simulink model "psbturbine"  (Simulink 6.0)
settings: Solver=ode23tb  SolverMode=SingleTasking  StartTime=0.0  StopTime=2  RelTol=1e-3
undefined symbols (not defined in the file or in its folder): D1, Delta
libraries: powerlib2 x15
settings Model: Creator=patrice  LastModifiedBy=batserve  ExtModeTrigMode=oneshot  ExtModeArmWhenConnect=off  ExtModeAutoUpdateStatusClock=off
settings DataIOCC: LimitDataPoints=off  SignalLoggingName=sigsOut
settings OptimizationCC: BlockReduction=off  BooleanDataType=off
settings DebuggingCC: CheckExecutionContextPreStartOutputMsg=on  CheckExecutionContextRuntimeOutputMsg=on  SolverPrmCheckMsg=none
settings HardwareCC: TargetUnknown=on
settings RTWCC: TemplateMakefile=grt_unix.tmf

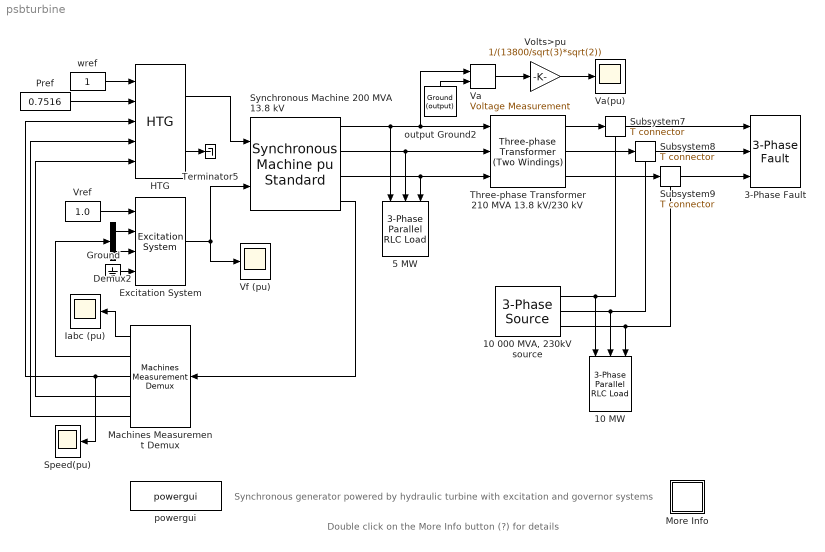
== system psbturbine ==
  note: Double click on the More Info button (?) for details
  note: Synchronous generator powered by hydraulic turbine
      |  with excitation and governor systems
  " Iabc (pu)" : Scope
      settings: TickLabels=on  TimeRange=0.2  YMax=6  DataFormat=Array
  " Speed(pu)" : Scope
      settings: TickLabels=on  TimeRange=2  YMin=0.98  YMax=1.02  SaveName=Pm  DataFormat=Array
  "10 000 MVA, 230kV source" : powerlib2/Electrical Sources/3-Phase Source  Tag=PoWeRsYsTeMbLoCk  V=230e3  Phi=0  F=60  InternalConnection=Yg  RLoff=on  R=0.529  L=0.0140  Psc=10000e6  Vbase=230e3  XRratio=10  PSBOutputType=111
  10 MW : powerlib2/Elements/3-Phase Parallel RLC Load  Orientation=down  Vpp=230e3  fn=60  P3=10e6  QL3=0  QC3=0
  3-Phase Fault : powerlib2/Elements/3-Phase Fault  sa=on  sb=on  sc=on  Rdef=1e-3  st=on  Rt=1e-3  comext=off  sw_status=[1 0]  sw_times=[ 0.1 0.2]  Ts=0  init_statext=[1 1 0]  Rp=inf  Cp=inf  mesure=None
  5 MW : powerlib2/Elements/3-Phase Parallel RLC Load  Orientation=down  Vpp=13.8e3  fn=60  P3=5e6  QL3=0  QC3=0
  Demux2 : Demux  Outputs=2
  Excitation System : powerlib2/Machines/Excitation System  tr=20e-3  reg=[ 300, 0.001 ]  exc=[ 1, 0 ]  tgr=[ 0, 0 ]  damp=[ 0.001, 0.1 ]  sat=[ 0, 0 ]  lim=[ -11.5, 11.5, 0 ]  v0=[1,1.0]
  Ground : Ground
  HTG : powerlib2/Machines/HTG  sm="[ 10/3  0.07 ]"  gate="[  0.01  0.97518  -0.1  0.1 ]"  reg="[  0.05  1.163  0.105  0  0.01  ]"  hyd="[  0  2.67  ]"  dref=0  po=1
  Machines Measurement Demux : powerlib2/Machines/Machines Measurement Demux  Orientation=left  machType=Synchronous  ssm1=on  ssm2=on  ssm3=on  ssm4=on  ssm5=on  ssm6=on  sm1=on  sm2=off  sm3=off  sm4=off  sm5=off  sm6=on  sm7=off  sm8=on  sm9=off  sm10=on  sm11=off  sm115=off  sm12=off  sm13=on  sm14=off  asm1=on  asm2=on  asm3=on  asm4=on  asm5=on  asm6=on  asm7=on  asm8=on  asm9=on  asm10=on  asm11=on  pmsm1=on  pmsm2=on  pmsm3=on  pmsm4=on  pmsm5=on  pmsm6=on  lastType=2
  More Info : Subsystem
      mask Display: disp('?')
  Pref : Constant  Value=0.7516
  Subsystem7 : powerlib2/Connectors/T connector  Tag=PoWeRsYsTeMbLoCk  PSBOutputType=1
  Subsystem8 : powerlib2/Connectors/T connector  Tag=PoWeRsYsTeMbLoCk  PSBOutputType=1
  Subsystem9 : powerlib2/Connectors/T connector  Tag=PoWeRsYsTeMbLoCk  PSBOutputType=1
  Synchronous Machine 200 MVA 13.8 kV : powerlib2/Machines/Synchronous Machine pu Standard  Tag=PoWeRsYsTeMbLoCk  rotorType=Salient-pole  x1="[ 200E6  13800   60 ]"  x2b=[ 31 32 33 34 35 36 37 ]  x2=[ 1.305, 0.296, 0.252, 0.474, 0.243, 0.18 ]  dAxisT=Short-circuit  qAxisT=Open-circuit  x3a=[]  x3b=[]  x3c=[]  x3d=[]  x3=[ 1.01, 0.053, 0.1 ]  x3e=[]  x3f=[]  x3g=[]  x4=2.8544e-3  x5="[ 3.2 0  32]"  x6=[0 0 0 0 0 0 0 0 1]  x7=off  x8=[0.6404,0.7127,0.8441,0.9214,0.9956,1.082,1.19,1.316,1.457;0.7,0.7698,0.8872,0.9466,0.9969,1.046,1.1,1.151,1.201]  PSBOutputType=1110  iounits=0.5  LoadFlowParameters=[1 150000000 0 0]
  Terminator5 : Terminator
  Three-phase Transformer 210 MVA 13.8 kV/230 kV : powerlib2/Elements/Three-phase Transformer (Two Windings)  Tag=PoWeRsYsTeMbLoCk  nominal=[ 210e6 60 ]  type1=Delta (D1)  params1="[ 13.8e3 0.0027  0.08]"  type2=Yg  params2=[ 230e3 0.0027 0.08]  ynsat=off  rmag=500  lm=500  sat="[ 0,0  ;  0.005,1.2  ;  1.0,1.4 ]"  hyst=off  matfile='hysteresis'  sif=off  phi0=[ 0.8 , -0.8 , 0.7 ]  initialslopes=[+1 +1 +1]  mesure=None  PSBOutputType=1111
  Va : powerlib2/Measurements/Voltage Measurement  Tag=PoWeRsYsTeMmEaSuReMeNt  PhasorSimulation=off  OutputType=Magnitude  PSBOutputType=0  PSBequivalent=0
  Va(pu) : Scope
      settings: TickLabels=on  TimeRange=0.2  YMin=-1.25  YMax=1.25  SaveName=vf  DataFormat=Array
  Vf (pu) : Scope
      settings: TickLabels=on  TimeRange=2  YMin=-10  YMax=15  SaveName=vf  DataFormat=Array
  Volts>pu : Gain  Gain=1/(13800/sqrt(3)*sqrt(2))  SaturateOnIntegerOverflow=on
  Vref : Constant  Value=1.0
  output Ground2 : powerlib2/Connectors/Ground (output)  Tag=PoWeRsYsTeMbLoCk  Orientation=up  PSBOutputType=1
  powergui : powerlib2/powergui  Frange=logspace(0,3,50)  Ylog=off  Xlog=off  save=off  variable=ZData  ZoomFFT=on  StartTime=0.0  cycles=2  DisplayStyle=off  fundamental=60  FreqAxis=off  MaxFrequency=1000  frequencyindice=1  frequencyindicesteady=1  RmsSteady=1  display=off  Ts=0  methode=off  frequency=60  echomessages=off
  wref : Constant
  wires:
  Ground/1 -> Excitation System/4
  HTG/2 -> Terminator5/1
  Excitation System/1 -> Vf (pu)/1, Synchronous Machine 200 MVA 13.8 kV/2
  Vref/1 -> Excitation System/1
  HTG/1 -> Synchronous Machine 200 MVA 13.8 kV/1
  Pref/1 -> HTG/2
  wref/1 -> HTG/1
  Machines Measurement Demux/1 -> " Iabc (pu)"/1
  Synchronous Machine 200 MVA 13.8 kV/4 -> Machines Measurement Demux/1
  "10 000 MVA, 230kV source"/3 -> 10 MW/3, Subsystem9/Enable
  "10 000 MVA, 230kV source"/2 -> 10 MW/2, Subsystem8/Enable
  "10 000 MVA, 230kV source"/1 -> 10 MW/1, Subsystem7/Enable
  Volts>pu/1 -> Va(pu)/1
  Va/1 -> Volts>pu/1
  output Ground2/1 -> Va/2
  Subsystem9/1 -> 3-Phase Fault/3
  Subsystem8/1 -> 3-Phase Fault/2
  Subsystem7/1 -> 3-Phase Fault/1
  Three-phase Transformer 210 MVA 13.8 kV/230 kV/3 -> Subsystem9/1
  Three-phase Transformer 210 MVA 13.8 kV/230 kV/2 -> Subsystem8/1
  Three-phase Transformer 210 MVA 13.8 kV/230 kV/1 -> Subsystem7/1
  Synchronous Machine 200 MVA 13.8 kV/3 -> 5 MW/3, Three-phase Transformer 210 MVA 13.8 kV/230 kV/3
  Synchronous Machine 200 MVA 13.8 kV/2 -> 5 MW/2, Three-phase Transformer 210 MVA 13.8 kV/230 kV/2
  Synchronous Machine 200 MVA 13.8 kV/1 -> Va/1, Three-phase Transformer 210 MVA 13.8 kV/230 kV/1, 5 MW/1
  Demux2/1 -> Excitation System/2
  Demux2/2 -> Excitation System/3
  Machines Measurement Demux/2 -> Demux2/1
  Machines Measurement Demux/4 -> HTG/5
  Machines Measurement Demux/3 -> HTG/3, " Speed(pu)"/1
  Machines Measurement Demux/5 -> HTG/4

== system psbturbine/More Info ==
  note: 4
  note: In order to start the simulation in steady state with the HTG and excitation system connected,  these two Simulink blocks must also be initialized
      | according to the values calculated by the load flow. This initialization is automatically performed when you execute the Load Flow, as long as you connect  at
      | the Pm and Vf inputs of the machine either Constant blocks or regulation blocks from the machine library (HTG, STG, or Excitation System).
      | Open the HTG block menu and notice that the initial mechanical  power has been automatically set to 0.5007 pu (100.14 MW) by the Load Flow.
      | Then, open the Excitation System block menu and note that the initial terminal voltage and field voltage have been set respectively to 1.0 and 1.1291 pu.
  note: 2
  note: Start Simulation and observe the three machine currents on the Iabc scope. If  the 9 parameters defining initial conditions
      | for the Synchronous Machine are set at zero or not set correctly , the simulation will not start in steady state.
  note: A three-phase generator rated 200 MVA, 13.8 kV, 112.5 rpm is connected to a 230 kV, 10 000 MVA network  through a Delta-Wye 210 MVA transformer.
      | At t = 0.1 s, a three-phase to ground fault occurs on the 230 kV bus. The fault is cleared after 6 cycles (t = 0.2 s).
      | During this demo, you will initialize the system in order to start in steady-state with the generator  supplying 150 MW of active power
      | and observe the dynamic response of the machine and of its voltage and speed regulators.
  note: This demonstration illustrates use of the synchronous machine associated with
      | the Hydraulic Turbine and Governor (HTG) and Excitation System blocks and use of
      | the Load Flow to initialize machine currents
  note: Circuit Description
  note: Demonstration
  note: 1
  note: 3
  note: Open the 4 scopes  and restart the simulation. The simulation now starts in steady state.
      | Observe that the terminal voltage Va is 1.0 p.u. at the beginning of the simulation. It falls to about 0.4 pu during the fault and returns to nominal
      | quickly after the fault is cleared. This quick response in terminal voltage is due to the fact that the Excitation System output Vf can go as high as 11.5 pu
      | which it does during the fault. The speed of the machine  increases to 1.01 pu during the fault then  it oscillates around 1 p.u. as the governor system regulates it.
      | The speed takes much  longer than the terminal voltage to stabilize mainly because the rate of valve opening/closing in the governor system is limited to 0.1 pu/s.
  note: In order to start the simulation in steady-state you must initialize the synchronous machine for the desired load flow.
      | Open the Powergyu and select 'Load Flow and Machine Initialization' . A new window appears. The machine 'Bus type' should be already initialized as
      | 'PV generator', indicating that  the load flow will be performed with the machine controlling the active power and its terminal voltage.
      | Specify the desired values by entering  the following parameters :
  note: Louis-A. Dessaint and R. Champagne (Ecole de Technologie Superieure, Montreal)
  note: Once the load flow has been solved the phasors of AB and BC machine voltages as well as the currents flowing out of phases A and B are updated.
      | The machine reactive power,  mechanical power and  field voltage requested to supply the electrical power should also be displayed:
      | Q = 3.4 Mvar; Pmec = 150.32 MW (0.7516 pu) ; field voltage Ef = 1.291 pu;
  note: Load flow : Terminal voltage (Vrms) = 13800; Active Power = 150e6. Then press the 'Execute Load Flow' button.
